simulink model "igrf_test"  (R2023a)
settings: Solver=VariableStepDiscrete  StartTime=0.0  StopTime=6000  MaxStep=1  RelTol=1e-3  EnableMultiTasking=on
libraries: aausat3_lib x7
settings Model: Creator=kasperv  LastModifiedBy=jacobel-omar
settings SolverCC: AlgebraicLoopSolver=TrustRegion
settings DataIOCC: LimitDataPoints=on  SaveFormat=Array  SignalLoggingSaveFormat=ModelDataLogs  ReturnWorkspaceOutputs=off
settings OptimizationCC: ExpressionDepthLimit=2147483647  LifeSpan=inf
settings DebuggingCC: UnderspecifiedInitializationDetection=Classic  MergeDetectMultiDrivingBlocksExec=none  SolverPrmCheckMsg=warning  FcnCallInpInsideContextMsg=warning  UnconnectedInputMsg=warning  UnconnectedOutputMsg=warning  UnconnectedLineMsg=warning  StateNameClashWarn=warning  SFUnexpectedBacktrackingDiag=warning  SFNoUnconditionalDefaultTransitionDiag=warning  SFExecutionAtInitializationDiag=none  ArithmeticOperatorsInVariantConditions=warning
settings HardwareCC: ProdBitPerPointer=32  ProdBitPerSizeT=32  ProdBitPerPtrDiffT=32  ProdLargestAtomicInteger=Long  ProdIntDivRoundTo=Undefined  ProdWordSize=32  ProdHWDeviceType=ARM Compatible->ARM 7
settings ModelReferenceCC: PropagateSignalLabelsOutOfModel=off
settings SFSimCC: SimUseLocalCustomCode=off  CustomCodeUndefinedFunction=UseInterfaceOnly
settings RTWCC: RTWUseLocalCustomCode=off
settings CodeAppCC: StateflowObjectComments=on
settings GRTTargetCC: TargetLangStandard=C89/C90 (ANSI)  CombineOutputUpdateFcns=off  GRTInterface=on
settings ConfigComp: CovMetricSettings=dw  CovSaveCumulativeToWorkspaceVar=on  CovSaveSingleToWorkspaceVar=on  CovExternalEMLEnable=off

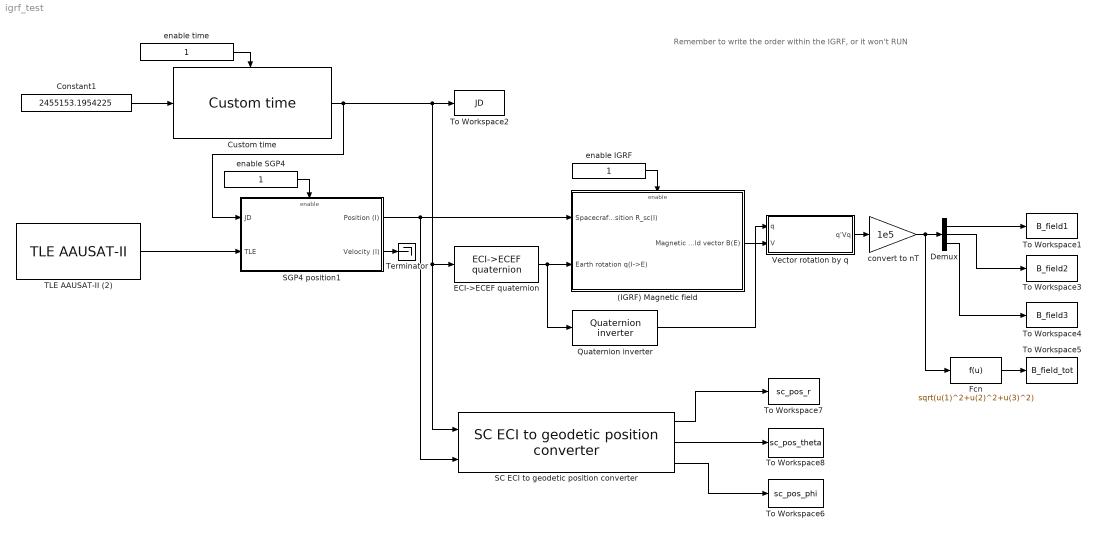
== system igrf_test ==
  note: Remember to write the order within the IGRF, or it won't RUN
  (IGRF) Magnetic field : Subsystem  AncestorBlock=aausat3_lib/Orbit and Ephemeris/(IGRF) Magnetic field  TreatAsAtomicUnit=on
  Constant1 : Constant  Value=2455153.1954225
  Custom time : aausat3_lib/Orbit and Ephemeris/Custom time  SystemSampleTime=-1  VariantActivationTime=update diagram  Latency=0  AutoFrameSizeCalculation=off
      settings: SourceProductName=AAUSAT3
  Demux : Demux  Outputs=3
  ECI->ECEF quaternion : aausat3_lib/Orbit and Ephemeris/ECI->ECEF quaternion  SystemSampleTime=-1  VariantActivationTime=update diagram  Latency=0  AutoFrameSizeCalculation=off
      settings: SourceProductName=AAUSAT3
  Fcn : Fcn  Expr=sqrt(u(1)^2+u(2)^2+u(3)^2)
  Quaternion inverter : aausat3_lib/Math Utilities/Quaternion operations/Quaternion inverter  SystemSampleTime=-1  VariantActivationTime=update diagram  Latency=0  AutoFrameSizeCalculation=off
      settings: SourceProductName=AAUSAT3
  SC ECI to geodetic position converter : aausat3_lib/Other Model Utilities/SC ECI to geodetic position converter
      settings: SourceProductName=AAUSAT3
  SGP4 position1 : Subsystem  AncestorBlock=aausat3_lib/Orbit and Ephemeris/SGP4 position  TreatAsAtomicUnit=on
  TLE AAUSAT-II (2) : aausat3_lib/Orbit and Ephemeris/TLE AAUSAT-II  satname='AAUSAT-II'  JulianDay=09321.69542252  xndt2o=0.00000555  xndd6o=0.0  bstar=.76898e-4  xincl=97.9251  xnodeo=24.1597  eo=0.0014245  omegao=254.1774  xmo=105.7862  xno=14.81823818  ts=1
      settings: SourceProductName=AAUSAT3
  Terminator : Terminator
  To Workspace1 : ToWorkspace  VariableName=B_field1  SampleTime=-1
  To Workspace2 : ToWorkspace  VariableName=JD  SampleTime=-1
  To Workspace3 : ToWorkspace  VariableName=B_field2  SampleTime=-1
  To Workspace4 : ToWorkspace  VariableName=B_field3  SampleTime=-1
  To Workspace5 : ToWorkspace  VariableName=B_field_tot  SampleTime=-1
  To Workspace6 : ToWorkspace  VariableName=sc_pos_phi  SampleTime=-1
  To Workspace7 : ToWorkspace  VariableName=sc_pos_r  SampleTime=-1
  To Workspace8 : ToWorkspace  VariableName=sc_pos_theta  SampleTime=-1
  Vector rotation by q : Subsystem  AncestorBlock=aausat3_lib/Math Utilities/Quaternion operations/Vector rotation by q
  convert to nT : Gain  Gain=1e5
  enable IGRF : Constant
  enable SGP4 : Constant
  enable time : Constant
  wires:
  convert to nT/1 -> Fcn/1, Demux/1
  (IGRF) Magnetic field/1(Magnetic field vector B(E)) -> Vector rotation by q/2(V)
  enable SGP4/1 -> SGP4 position1/Enable
  Custom time/1 -> To Workspace2/1, ECI->ECEF quaternion/1, SC ECI to geodetic position converter/1, SGP4 position1/1(JD)
  enable time/1 -> Custom time/Enable
  Quaternion inverter/1 -> Vector rotation by q/1(q)
  Vector rotation by q/1(q'Vq) -> convert to nT/1
  SGP4 position1/1(Position (I)) -> (IGRF) Magnetic field/1(Spacecraft position R_sc(I)), SC ECI to geodetic position converter/2
  ECI->ECEF quaternion/1 -> (IGRF) Magnetic field/2(Earth rotation q(I->E)), Quaternion inverter/1
  SGP4 position1/2(Velocity (I)) -> Terminator/1
  Fcn/1 -> To Workspace5/1
  enable IGRF/1 -> (IGRF) Magnetic field/Enable
  TLE AAUSAT-II (2)/1 -> SGP4 position1/2(TLE)
  Constant1/1 -> Custom time/1
  Demux/3 -> To Workspace4/1
  Demux/2 -> To Workspace3/1
  Demux/1 -> To Workspace1/1
  SC ECI to geodetic position converter/2 -> To Workspace8/1
  SC ECI to geodetic position converter/1 -> To Workspace7/1
  SC ECI to geodetic position converter/3 -> To Workspace6/1

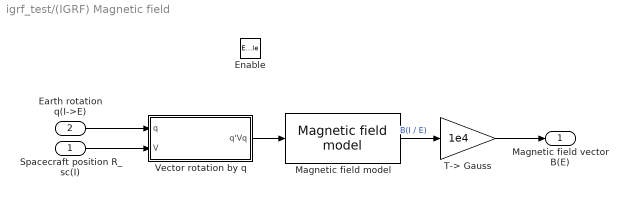
== system igrf_test/(IGRF) Magnetic field ==
  Spacecraft position R_sc(I) : Inport
  Earth rotation q(I->E) : Inport  Port=2
  Enable : EnablePort
  Magnetic field model : aausat3_lib/Orbit and Ephemeris/Magnetic field model  SystemSampleTime=-1  VariantActivationTime=update diagram  Latency=0  AutoFrameSizeCalculation=off
      link override S-Function: Parameters=2009.88,order
      settings: SourceProductName=AAUSAT3
  T-> Gauss : Gain  Gain=1e4
  Vector rotation by q : Subsystem  AncestorBlock=aausat3_lib/Math Utilities/Quaternion operations/Vector rotation by q
  Magnetic field vector B(E) : Outport
  wires:
  Spacecraft position R_sc(I)/1 -> Vector rotation by q/2(V)
  Earth rotation q(I->E)/1 -> Vector rotation by q/1(q)
  Vector rotation by q/1(q'Vq) -> Magnetic field model/1
  Magnetic field model/1 -> T-> Gauss/1  "B(I / E)"
  T-> Gauss/1 -> Magnetic field vector B(E)/1

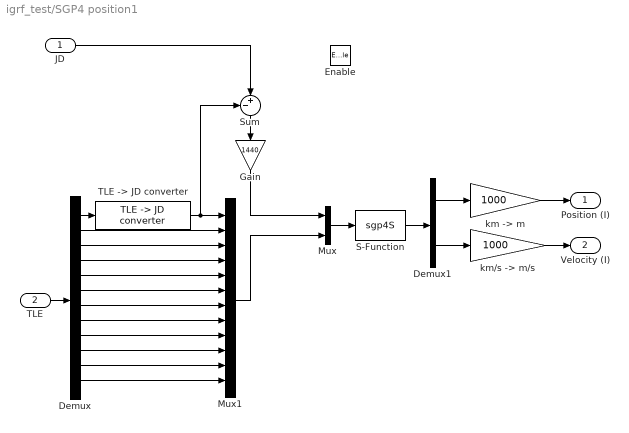
== system igrf_test/SGP4 position1 ==
  JD : Inport
  TLE : Inport  Port=2
  Enable : EnablePort
  " S-Function" : S-Function  FunctionName=sgp4S  SFunctionDeploymentMode=off  EnableBusSupport=off
  Demux : Demux  Outputs=12
  Demux1 : Demux  Outputs=[3 3]
      settings: DisplayOption=none
  Gain : Gain  Gain=1440
  Mux : Mux  Inputs=2
  Mux1 : Mux  Inputs=12
  Sum : Sum  Inputs=-+|  InputSameDT=on  SaturateOnIntegerOverflow=on  OutDataTypeStr=Inherit: Same as first input
  "TLE -> JD converter" : aausat3_lib/Other Model Utilities/TLE -> JD converter  SystemSampleTime=-1  VariantActivationTime=update diagram  Latency=0  AutoFrameSizeCalculation=off
      settings: SourceProductName=AAUSAT3
  "km -> m" : Gain  Gain=1000  SaturateOnIntegerOverflow=on  OutDataTypeStr=Inherit: Same as input  ParamDataTypeStr=Inherit: Same as input
  "km/s -> m/s" : Gain  Gain=1000  SaturateOnIntegerOverflow=on  OutDataTypeStr=Inherit: Same as input  ParamDataTypeStr=Inherit: Same as input
  Position (I) : Outport  InitialOutput=0
  Velocity (I) : Outport  Port=2  InitialOutput=0
  wires:
  JD/1 -> Sum/2
  "km -> m"/1 -> Position (I)/1
  "km/s -> m/s"/1 -> Velocity (I)/1
  Mux/1 -> " S-Function"/1
  " S-Function"/1 -> Demux1/1
  Demux1/2 -> "km/s -> m/s"/1
  Demux1/1 -> "km -> m"/1
  TLE/1 -> Demux/1
  Demux/2 -> Mux1/2
  Demux/3 -> Mux1/3
  Demux/4 -> Mux1/4
  Demux/5 -> Mux1/5
  Demux/6 -> Mux1/6
  Demux/7 -> Mux1/7
  Demux/8 -> Mux1/8
  Demux/9 -> Mux1/9
  Demux/10 -> Mux1/10
  Demux/11 -> Mux1/11
  Demux/12 -> Mux1/12
  Mux1/1 -> Mux/2
  Demux/1 -> "TLE -> JD converter"/1
  "TLE -> JD converter"/1 -> Mux1/1, Sum/1
  Sum/1 -> Gain/1
  Gain/1 -> Mux/1

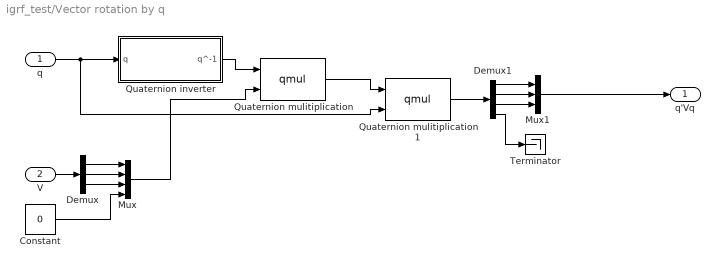
== system igrf_test/Vector rotation by q ==
  q : Inport
  V : Inport  Port=2
  Constant : Constant  Value=0
  Demux : Demux  Outputs=3
      settings: DisplayOption=none
  Demux1 : Demux
      settings: DisplayOption=none
  Mux : Mux
  Mux1 : Mux  Inputs=3
  Quaternion inverter : Subsystem
  Quaternion mulitiplication : S-Function  FunctionName=qmul  SFunctionDeploymentMode=off  EnableBusSupport=off
  Quaternion mulitiplication1 : S-Function  FunctionName=qmul  SFunctionDeploymentMode=off  EnableBusSupport=off
  Terminator : Terminator
  q'Vq : Outport
  wires:
  Mux1/1 -> q'Vq/1
  Demux1/4 -> Terminator/1
  Demux1/3 -> Mux1/3
  Demux1/2 -> Mux1/2
  Demux1/1 -> Mux1/1
  Quaternion mulitiplication1/1 -> Demux1/1
  Quaternion mulitiplication/1 -> Quaternion mulitiplication1/1
  Mux/1 -> Quaternion mulitiplication/2
  Constant/1 -> Mux/4
  Demux/3 -> Mux/3
  Demux/2 -> Mux/2
  Demux/1 -> Mux/1
  V/1 -> Demux/1
  q/1 -> Quaternion inverter/1(q), Quaternion mulitiplication1/2
  Quaternion inverter/1(q^-1) -> Quaternion mulitiplication/1

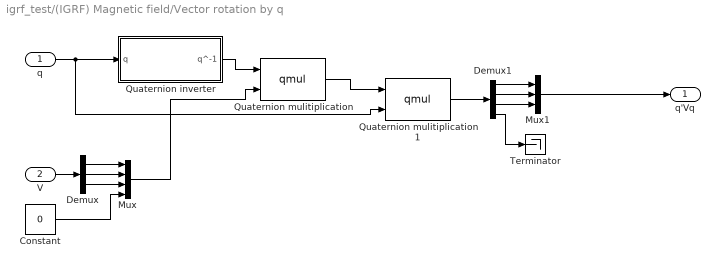
== system igrf_test/(IGRF) Magnetic field/Vector rotation by q ==
  q : Inport
  V : Inport  Port=2
  Constant : Constant  Value=0
  Demux : Demux  Outputs=3
      settings: DisplayOption=none
  Demux1 : Demux
      settings: DisplayOption=none
  Mux : Mux
  Mux1 : Mux  Inputs=3
  Quaternion inverter : Subsystem
  Quaternion mulitiplication : S-Function  FunctionName=qmul  SFunctionDeploymentMode=off  EnableBusSupport=off
  Quaternion mulitiplication1 : S-Function  FunctionName=qmul  SFunctionDeploymentMode=off  EnableBusSupport=off
  Terminator : Terminator
  q'Vq : Outport
  wires:
  Mux1/1 -> q'Vq/1
  Demux1/4 -> Terminator/1
  Demux1/3 -> Mux1/3
  Demux1/2 -> Mux1/2
  Demux1/1 -> Mux1/1
  Quaternion mulitiplication1/1 -> Demux1/1
  Mux/1 -> Quaternion mulitiplication/2
  Constant/1 -> Mux/4
  Demux/3 -> Mux/3
  Demux/2 -> Mux/2
  Demux/1 -> Mux/1
  V/1 -> Demux/1
  q/1 -> Quaternion inverter/1(q), Quaternion mulitiplication1/2
  Quaternion mulitiplication/1 -> Quaternion mulitiplication1/1
  Quaternion inverter/1(q^-1) -> Quaternion mulitiplication/1

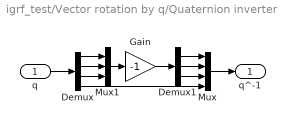
== system igrf_test/Vector rotation by q/Quaternion inverter ==
  q : Inport
  Demux : Demux
      settings: DisplayOption=none
  Demux1 : Demux  Outputs=3
      settings: DisplayOption=none
  Gain : Gain  Gain=-1  SaturateOnIntegerOverflow=on  OutDataTypeStr=Inherit: Same as input  ParamDataTypeStr=Inherit: Same as input
  Mux : Mux
  Mux1 : Mux  Inputs=3
  q^-1 : Outport
  wires:
  Gain/1 -> Demux1/1
  Demux1/3 -> Mux/3
  Demux1/2 -> Mux/2
  Demux1/1 -> Mux/1
  Mux1/1 -> Gain/1
  Demux/3 -> Mux1/3
  Demux/2 -> Mux1/2
  Demux/1 -> Mux1/1
  Demux/4 -> Mux/4
  Mux/1 -> q^-1/1
  q/1 -> Demux/1

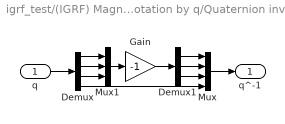
== system igrf_test/(IGRF) Magnetic field/Vector rotation by q/Quaternion inverter ==
  q : Inport
  Demux : Demux
      settings: DisplayOption=none
  Demux1 : Demux  Outputs=3
      settings: DisplayOption=none
  Gain : Gain  Gain=-1  SaturateOnIntegerOverflow=on  OutDataTypeStr=Inherit: Same as input  ParamDataTypeStr=Inherit: Same as input
  Mux : Mux
  Mux1 : Mux  Inputs=3
  q^-1 : Outport
  wires:
  Gain/1 -> Demux1/1
  Demux1/3 -> Mux/3
  Demux1/2 -> Mux/2
  Demux1/1 -> Mux/1
  Mux1/1 -> Gain/1
  Demux/3 -> Mux1/3
  Demux/2 -> Mux1/2
  Demux/1 -> Mux1/1
  Demux/4 -> Mux/4
  Mux/1 -> q^-1/1
  q/1 -> Demux/1
